simulink model "sim_full"  (R2020a)
settings: Solver=VariableStepAuto  StartTime=0.0  StopTime=10.0  RelTol=1e-3
values from neighbouring files (symbols this model uses):
  buffer = 0.0    (= 0)    [a_1.m]    (also in a_2.m; a_loss_function.m; full_model.m; part2.m)
  gov = 0.5    [a_1.m]    (also in a_2.m; a_loss_function.m; bank_centralbank.m; full_model.m)
  hike = 0.0    (= 0)    [a_1.m]    (also in a_2.m = 0.01; a_loss_function.m; full_model.m; part2.m = 0.01)
  i_cb = 0.03    [a_1.m]    (also in a_2.m = 0.07; a_loss_function.m; full_model.m; part2.m = 0.1)
  i_diff = 0.025    [a_1.m]    (also in a_2.m; a_loss_function.m; bank_and_economy.m = 0.02; full_model.m)
  i_k = 0.06    [a_1.m]    (also in a_loss_function.m = 0.04; bank_and_economy.m = 0.04; full_model.m = 0.04)
  K_0 = 0.08    [a_1.m]    (also in a_2.m; a_loss_function.m; bank_and_economy.m; bank_centralbank.m)
  K_p = 15    [a_1.m]    (also in a_2.m; a_loss_function.m; bank_and_economy.m = 0.5; bank_centralbank.m)
  lambda = 0.002    [a_1.m]    (also in a_2.m; a_loss_function.m; bank_and_economy.m; bank_centralbank.m)
  lambda_k = 0.005    [a_1.m]    (also in a_2.m; a_loss_function.m; full_model.m; part2.m)
  R = 1    [a_1.m]    (also in a_2.m; a_loss_function.m; bank_and_economy.m; bank_centralbank.m)
  r_k = 0.1    [a_1.m]    (also in a_2.m; a_loss_function.m; bank_and_economy.m; full_model.m)
  rate = 0.1    [a_1.m]    (also in a_2.m; a_loss_function.m; bank_and_economy.m; bank_centralbank.m)
  re = 0.3    [a_1.m]    (also in a_2.m; a_loss_function.m; full_model.m; part2.m)
  sigma = 0.28    [a_1.m]    (also in a_2.m; a_loss_function.m; bank_and_economy.m; bank_centralbank.m)
  sigma_k = 0.25    [a_loss_function.m]    (also in full_model.m)
  T_f = 0.5    [a_1.m]    (also in a_2.m; a_loss_function.m; bank_and_economy.m; bank_centralbank.m)
  T_g = 1    [a_1.m]    (also in a_2.m; a_loss_function.m; bank_and_economy.m; bank_centralbank.m)
  T_h = 0.1    [a_1.m]    (also in a_2.m; a_loss_function.m; bank_and_economy.m; bank_centralbank.m)
  T_i = 8    [a_1.m]    (also in a_2.m; a_loss_function.m; bank_and_economy.m; bank_centralbank.m)
  T_k = 0.1    [a_1.m]    (also in a_2.m; a_loss_function.m; bank_and_economy.m = 0.25; economy.m = 1)
  tx = 0.3    [a_1.m]    (also in a_2.m; a_loss_function.m; bank_and_economy.m = 0.5; bank_centralbank.m = 0.25)
  w = 0.4    [a_1.m]    (also in a_2.m; a_loss_function.m; full_model.m = 0.7; part2.m)
settings Model: Creator=erlended  LastModifiedBy=erlended

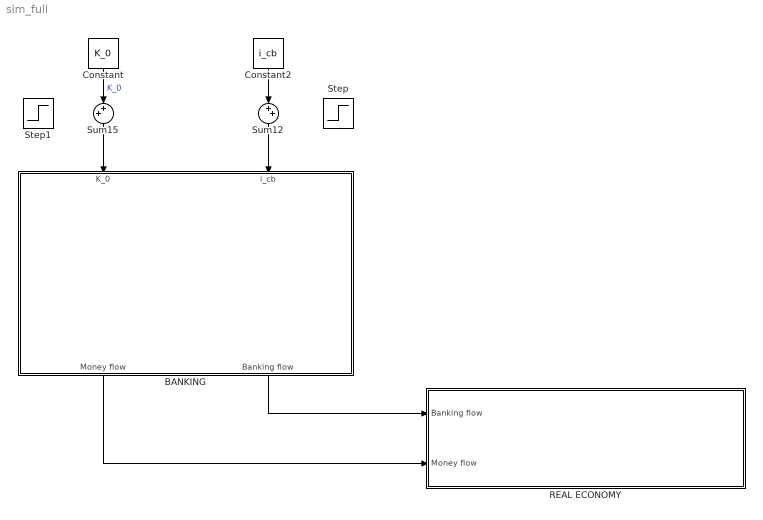
== system sim_full ==
  BANKING : Subsystem
  Constant : Constant  Value=K_0
  Constant2 : Constant  Value=i_cb
  REAL ECONOMY : Subsystem
  Step : Step  Time=10  After=hike  SampleTime=0
  Step1 : Step  Time=10  After=buffer  SampleTime=0
  Sum12 : Sum  Inputs=|++
  Sum15 : Sum  Inputs=++|
  wires:
  Constant2/1 -> Sum12/1
  Constant/1 -> Sum15/2  "K_0"
  Sum15/1 -> BANKING/1(K_0)
  BANKING/2(Banking flow) -> REAL ECONOMY/1(Banking flow)
  BANKING/1(Money flow) -> REAL ECONOMY/2(Money flow)
  Sum12/1 -> BANKING/2(i_cb)

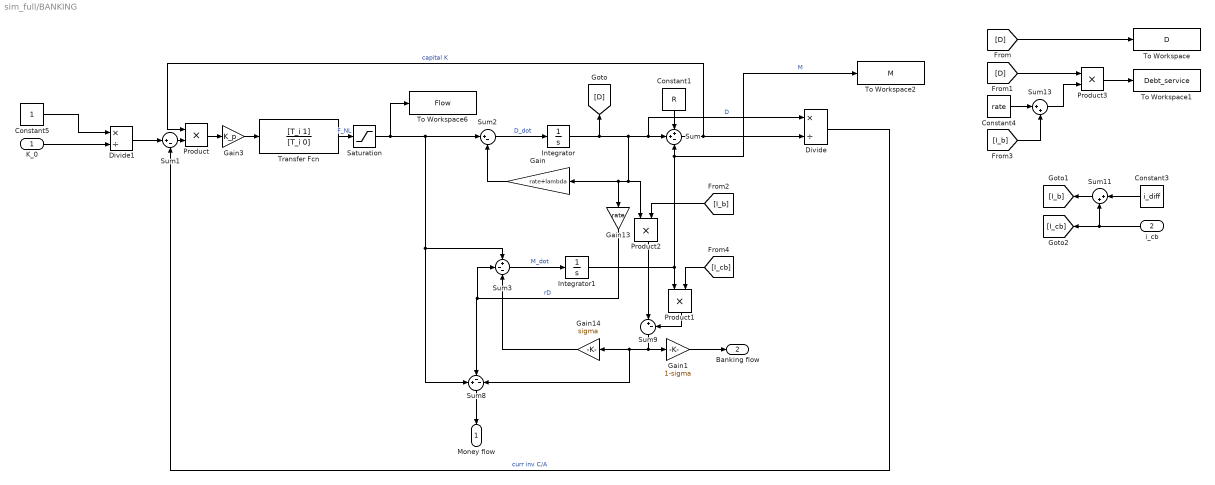
== system sim_full/BANKING ==
  K_0 : Inport
  i_cb : Inport  Port=2
  Constant1 : Constant  Value=R
  Constant3 : Constant  Value=i_diff
  Constant4 : Constant  Value=rate
  Constant5 : Constant
  Divide : Product  Inputs=*/
  Divide1 : Product  Inputs=*/
  Gain : Gain  Gain=rate+lambda
  Gain1 : Gain  Gain=1-sigma
  Gain13 : Gain  Gain=rate
  Gain14 : Gain  Gain=sigma
  Gain3 : Gain  Gain=K_p
  Integrator : Integrator
  Integrator1 : Integrator
  Product{,1..3} (4 alike) : Product
  Saturation : Saturate  UpperLimit=100  LowerLimit=0
  Sum : Sum  Inputs=++-
  Sum1 : Sum  Inputs=|+-
  Sum11 : Sum  Inputs=|++
  Sum13 : Sum  Inputs=|++
  Sum2 : Sum  Inputs=|+-
  Sum3 : Sum  Inputs=+--
  Sum8 : Sum  Inputs=+--
  Sum9 : Sum  Inputs=|+-
  To Workspace : ToWorkspace  VariableName=D  SaveFormat=Timeseries  SampleTime=-1
  To Workspace1 : ToWorkspace  VariableName=Debt_service  SaveFormat=Timeseries  SampleTime=-1
  To Workspace2 : ToWorkspace  VariableName=M  SaveFormat=Timeseries  SampleTime=-1
  To Workspace6 : ToWorkspace  VariableName=Flow  SaveFormat=Timeseries  SampleTime=-1
  Transfer Fcn : TransferFcn  Numerator=[T_i 1]  Denominator=[T_i 0]
  Money flow : Outport
  Banking flow : Outport  Port=2
  wires:
  Product/1 -> Gain3/1
  Integrator/1 -> Sum/2, Divide/1, Gain/1, Gain13/1, Product2/1, [D]  "D"
  Sum8/1 -> Money flow/1
  Integrator1/1 -> To Workspace2/1, Sum/3, Product1/1  "M"
  Saturation/1 -> Sum2/1, Sum3/1, Sum8/1, To Workspace6/1
  Transfer Fcn/1 -> Saturation/1  "F_NL"
  Sum/1 -> Product/1, Divide/2  "capital K"
  Gain/1 -> Sum2/2
  Gain13/1 -> Sum8/2, Sum3/2  "rD"
  Sum9/1 -> Gain1/1, Sum8/3, Gain14/1
  Sum2/1 -> Integrator/1  "D_dot"
  Constant3/1 -> Sum11/1
  Gain3/1 -> Transfer Fcn/1
  Constant1/1 -> Sum/1
  Divide/1 -> Sum1/2  "curr inv C/A"
  Sum1/1 -> Product/2
  Sum3/1 -> Integrator1/1  "M_dot"
  Constant4/1 -> Sum13/1
  Product2/1 -> Sum9/1
  Product1/1 -> Sum9/2
  Constant5/1 -> Divide1/1
  Product3/1 -> To Workspace1/1
  i_cb/1 -> [I_cb], Sum11/2
  Sum13/1 -> Product3/2
  Divide1/1 -> Sum1/1
  Gain14/1 -> Sum3/3
  Gain1/1 -> Banking flow/1
  K_0/1 -> Divide1/2
  [D] -> To Workspace/1
  [D] -> Product3/1
  Sum11/1 -> [I_b]
  [I_b] -> Product2/2
  [I_b] -> Sum13/2
  [I_cb] -> Product1/2

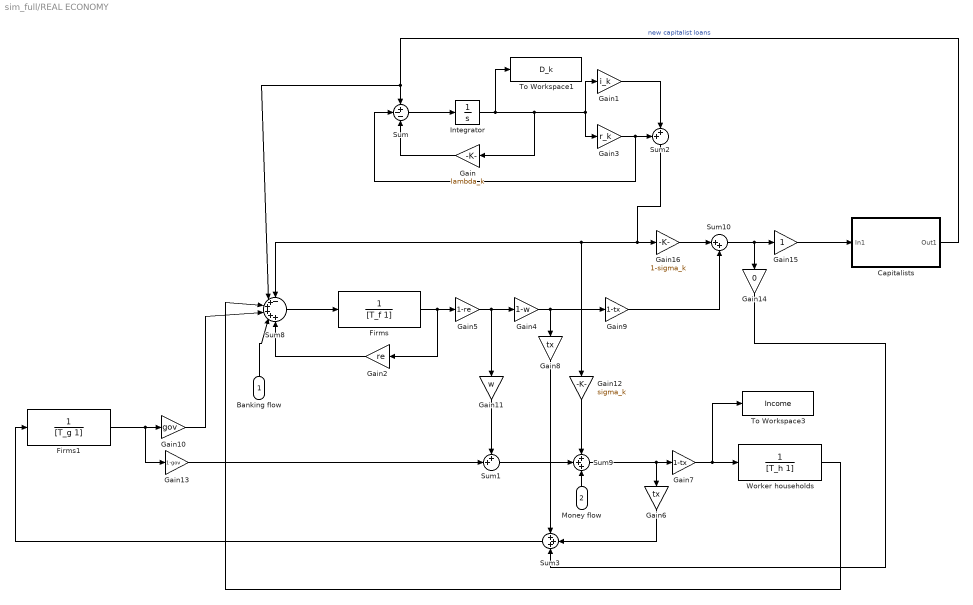
== system sim_full/REAL ECONOMY ==
  Banking flow : Inport
  Money flow : Inport  Port=2
  Capitalists : Subsystem
  Firms : TransferFcn  Denominator=[T_f 1]
  Firms1 : TransferFcn  Denominator=[T_g 1]
  Gain : Gain  Gain=lambda_k
  Gain1 : Gain  Gain=i_k
  Gain10 : Gain  Gain=gov
  Gain11 : Gain  Gain=w
  Gain12 : Gain  Gain=sigma_k
  Gain13 : Gain  Gain=1-gov
  Gain14 : Gain  Gain=0
  Gain15 : Gain
  Gain16 : Gain  Gain=1-sigma_k
  Gain2 : Gain  Gain=re
  Gain3 : Gain  Gain=r_k
  Gain4 : Gain  Gain=1-w
  Gain5 : Gain  Gain=1-re
  Gain6 : Gain  Gain=tx
  Gain7 : Gain  Gain=1-tx
  Gain8 : Gain  Gain=tx
  Gain9 : Gain  Gain=1-tx
  Integrator : Integrator
  Sum : Sum  Inputs=+--
  Sum1 : Sum  Inputs=++|
  Sum10 : Sum  Inputs=|++
  Sum2 : Sum  Inputs=++|
  Sum3 : Sum  Inputs=+++
  Sum8 : Sum  Inputs=-+++++
  Sum9 : Sum  Inputs=+++
  To Workspace1 : ToWorkspace  VariableName=D_k  SaveFormat=Timeseries  SampleTime=-1
  To Workspace3 : ToWorkspace  VariableName=Income  SaveFormat=Timeseries  SampleTime=-1
  Worker households : TransferFcn  Denominator=[T_h 1]
  wires:
  Worker households/1 -> Sum8/3
  Gain1/1 -> Sum2/2
  Sum8/1 -> Firms/1
  Firms/1 -> Gain2/1, Gain5/1
  Capitalists/1(Out1) -> Sum8/2, Sum/1  "new capitalist loans"
  Gain12/1 -> Sum9/1
  Integrator/1 -> Gain/1, Gain1/1, Gain3/1, To Workspace1/1
  Sum2/1 -> Sum8/1, Gain12/1, Gain16/1
  Gain16/1 -> Sum10/1
  Gain3/1 -> Sum/2, Sum2/1
  Sum/1 -> Integrator/1
  Gain/1 -> Sum/3
  Gain4/1 -> Gain8/1, Gain9/1
  Sum9/1 -> Gain7/1, Gain6/1
  Money flow/1 -> Sum9/3
  Gain5/1 -> Gain4/1, Gain11/1
  Sum3/1 -> Firms1/1
  Gain7/1 -> To Workspace3/1, Worker households/1
  Gain8/1 -> Sum3/1
  Gain6/1 -> Sum3/2
  Gain9/1 -> Sum10/2
  Firms1/1 -> Gain13/1, Gain10/1
  Gain11/1 -> Sum1/1
  Sum1/1 -> Sum9/2
  Gain13/1 -> Sum1/2
  Gain2/1 -> Sum8/6
  Banking flow/1 -> Sum8/5
  Gain10/1 -> Sum8/4
  Sum10/1 -> Gain14/1, Gain15/1
  Gain14/1 -> Sum3/3
  Gain15/1 -> Capitalists/1(In1)

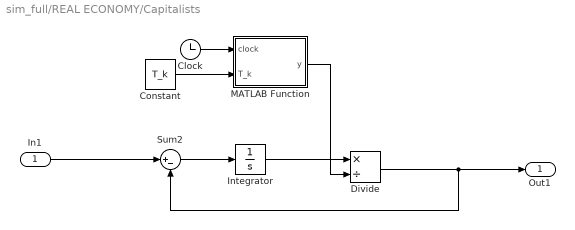
== system sim_full/REAL ECONOMY/Capitalists ==
  In1 : Inport
  Clock : Clock
  Constant : Constant  Value=T_k
  Divide : Product  Inputs=*/
  Integrator : Integrator
  MATLAB Function : MATLAB Function  TreatAsAtomicUnit=on
  Sum2 : Sum  Inputs=|+-
  Out1 : Outport
  wires:
  In1/1 -> Sum2/1
  Sum2/1 -> Integrator/1
  Divide/1 -> Out1/1, Sum2/2
  Integrator/1 -> Divide/1
  Clock/1 -> MATLAB Function/1(clock)
  MATLAB Function/1(y) -> Divide/2
  Constant/1 -> MATLAB Function/2(T_k)

== matlab function sim_full/REAL ECONOMY/Capitalists/MATLAB Function ==
  data: clock input; y output; T_k input
function y= fcn(clock, T_k)

if clock > 30
    y = 1;
else
    y = T_k;
end
